simulink library "avl2DLiftingBdy_cl"  (R2018b)
settings: Solver=VariableStepAuto  StartTime=0.0  StopTime=10.0  RelTol=1e-3
values from neighbouring files (symbols this model uses):
  Bref = 1    [avl2DLiftingBdy_ts.m]
  Cref = 1    [avl2DLiftingBdy_ts.m]
  grav = 9.81    [avl2DLiftingBdy_ts.m]
  mass = 10    [avl2DLiftingBdy_ts.m]
  Rcb_cm = [0;0;0.1]    [avl2DLiftingBdy_ts.m]
  rho_fluid = 1    [avl2DLiftingBdy_ts.m]
  Sref = 1    [avl2DLiftingBdy_ts.m]
  vol = 20    [avl2DLiftingBdy_ts.m]
undefined symbols (not defined in the file or in its folder): CDtot_2D_Tbl, class_thr, CLtot_2D_Tbl, Cltot_2D_Tbl, Cmtot_2D_Tbl, Cntot_2D_Tbl, ini_euler, ini_O_Vcm_o, ini_OwB, ini_Rcm_o, k_CS_gain, MI, turbine
libraries: BdyFrameGravForce_ul x1, avlAerodynamics2D x1, bdyFrameBuoyFnM_ul x1, calcTetherEndNodesStates x1, simpleDragTurbine_ul x1, sixDoFDynamics_ul x1, sumTetherForcesAndMoments_ul x1
settings Model: Creator=Ayaz  LastModifiedBy=Ayaz

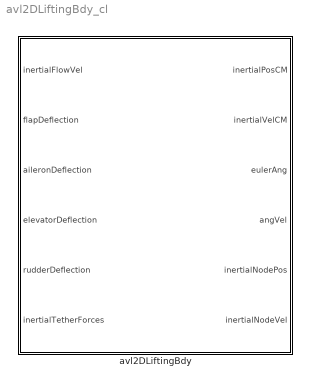
== system avl2DLiftingBdy_cl ==
  avl2DLiftingBdy : Subsystem  mask{M=mass, J=MI, vol=vol, Rcb_cm=Rcb_cm, turb_struct=turbine, thr_struct=class_thr, g=grav, rho_fluid=rho_fluid, initPos=ini_Rcm_o, initVel=ini_O_Vcm_o, initEulAngs=ini_euler, initAngVel=ini_OwB, CLTable=CLtot_2D_Tbl, CDTable=CDtot_2D_Tbl, CMxTable=Cltot_2D_Tbl, CMyTable=Cmtot_2D_Tbl, CMzTable=Cntot_2D_Tbl, CsGainMatrix=k_CS_gain, CRef=Cref, BRef=Bref, SRef=Sref}
      mask prompts: M "Mass"; J "Inertia matrix"; vol "Body volume"; Rcb_cm "Center of buoyamcy vector"; turb_struct "Turbines structure"; thr_struct "Tether class variable name"; g "Gravitational acceleration"; rho_fluid "Fluid density"; initPos "Initial position"; initVel "Initial velocity"; initEulAngs "Initial Euler Angles"; initAngVel "Initial Angular Velocity Vec"; CLTable "CL lookup table object"; CDTable "CD lookup table object"; CMxTable "CMx lookup table object"; CMyTable "CMy lookup table object"; CMzTable "CMz lookup table object"; CsGainMatrix "Control surface gain matrix"; CRef "Pitch Moment Reference Length (AVL Cref)"; BRef "Roll & Yaw Moment Reference Length (AVL Bref)"; SRef "Ref area (AVL Sref)"
      mask TypeOptions M: BdyFrameGravForce/M | sixDoFDynamics1/M
      mask TypeOptions J: sixDoFDynamics1/J
      mask TypeOptions vol: bdyFrameBuoyForceAndMoment/vol
      mask TypeOptions Rcb_cm: bdyFrameBuoyForceAndMoment/Rcb_cm
      mask TypeOptions turb_struct: simpleDragTurbine/turb_struct
      mask TypeOptions thr_struct: calcTetherEndNodesStates/thr_struct | sumTetherForcesAndMoments/thr_struct
      mask TypeOptions g: BdyFrameGravForce/g | bdyFrameBuoyForceAndMoment/g
      mask TypeOptions rho_fluid: avlAerodynamics2D/rho_fluid | bdyFrameBuoyForceAndMoment/rho_fluid | simpleDragTurbine/rho_fluid
      mask TypeOptions initPos: sixDoFDynamics1/initPos
      mask TypeOptions initVel: sixDoFDynamics1/initVel
      mask TypeOptions initEulAngs: sixDoFDynamics1/initEulAngs
      mask TypeOptions initAngVel: sixDoFDynamics1/initAngVel
      mask TypeOptions CLTable: avlAerodynamics2D/CLTable
      mask TypeOptions CDTable: avlAerodynamics2D/CDTable
      mask TypeOptions CMxTable: avlAerodynamics2D/CMxTable
      mask TypeOptions CMyTable: avlAerodynamics2D/CMyTable
      mask TypeOptions CMzTable: avlAerodynamics2D/CMzTable
      mask TypeOptions CsGainMatrix: avlAerodynamics2D/CsGainMatrix
      mask TypeOptions CRef: avlAerodynamics2D/CRef
      mask TypeOptions BRef: avlAerodynamics2D/BRef
      mask TypeOptions SRef: avlAerodynamics2D/SRef
      mask DialogControl Container20 Prompt: Parameters
      mask DialogControl ParameterGroupVar Prompt: Physical Parameters
      mask DialogControl Container24 Prompt: Environment
      mask DialogControl Container25 Prompt: Initial conditions
      mask DialogControl Container7 Prompt: AVL

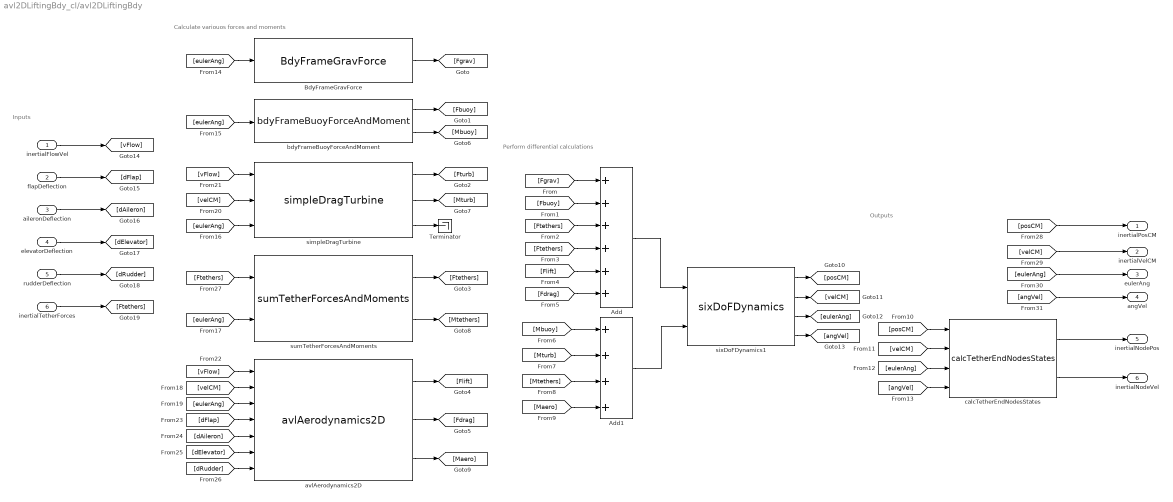
== system avl2DLiftingBdy_cl/avl2DLiftingBdy ==
  note: Outputs
  note: Inputs
  note: Calculate variouos forces and moments
  note: Perform differential calculations
  inertialFlowVel : Inport
  flapDeflection : Inport  Port=2
  aileronDeflection : Inport  Port=3
  elevatorDeflection : Inport  Port=4
  rudderDeflection : Inport  Port=5
  inertialTetherForces : Inport  Port=6
  Add : Sum  Inputs=++++++
  Add1 : Sum  Inputs=++++
  BdyFrameGravForce : BdyFrameGravForce_ul/BdyFrameGravForce  M=M  g=g
  Terminator : Terminator
  avlAerodynamics2D : avlAerodynamics2D/avlAerodynamics2D  CLTable=CLTable  CDTable=CDTable  CMxTable=CMxTable  CMyTable=CMyTable  CMzTable=CMzTable  CsGainMatrix=CsGainMatrix  CRef=CRef  BRef=BRef  SRef=SRef  rho_fluid=rho_fluid
  bdyFrameBuoyForceAndMoment : bdyFrameBuoyFnM_ul/bdyFrameBuoyForceAndMoment  vol=vol  rho_fluid=rho_fluid  g=g  Rcb_cm=Rcb_cm
  calcTetherEndNodesStates : calcTetherEndNodesStates/calcTetherEndNodesStates  thr_struct=thr_struct  attach_point=Lifting body
  simpleDragTurbine : simpleDragTurbine_ul/simpleDragTurbine  rho_fluid=rho_fluid  turb_struct=turb_struct
  sixDoFDynamics1 : sixDoFDynamics_ul/sixDoFDynamics  M=M  J=J  initPos=initPos  initVel=initVel  initEulAngs=initEulAngs  initAngVel=initAngVel
  sumTetherForcesAndMoments : sumTetherForcesAndMoments_ul/sumTetherForcesAndMoments  thr_struct=thr_struct  attach_point=Lifting body
  inertialPosCM : Outport
  inertialVelCM : Outport  Port=2
  eulerAng : Outport  Port=3
  angVel : Outport  Port=4
  inertialNodePos : Outport  Port=5
  inertialNodeVel : Outport  Port=6
  wires:
  [Mtethers] -> Add1/3
  [velCM] -> avlAerodynamics2D/2
  [angVel] -> calcTetherEndNodesStates/4
  [eulerAng] -> calcTetherEndNodesStates/3
  sixDoFDynamics1/4 -> [angVel]
  sixDoFDynamics1/3 -> [eulerAng]
  [posCM] -> calcTetherEndNodesStates/1
  sixDoFDynamics1/2 -> [velCM]
  [Mturb] -> Add1/2
  [eulerAng] -> sumTetherForcesAndMoments/2
  [eulerAng] -> bdyFrameBuoyForceAndMoment/1
  [eulerAng] -> BdyFrameGravForce/1
  [Mbuoy] -> Add1/1
  simpleDragTurbine/3 -> Terminator/1
  [Ftethers] -> Add/4
  avlAerodynamics2D/2 -> [Fdrag]
  Add1/1 -> sixDoFDynamics1/2
  avlAerodynamics2D/3 -> [Maero]
  [Fbuoy] -> Add/2
  avlAerodynamics2D/1 -> [Flift]
  sumTetherForcesAndMoments/1 -> [Ftethers]
  [velCM] -> calcTetherEndNodesStates/2
  [Maero] -> Add1/4
  [Ftethers] -> Add/3
  simpleDragTurbine/2 -> [Mturb]
  simpleDragTurbine/1 -> [Fturb]
  [Flift] -> Add/5
  Add/1 -> sixDoFDynamics1/1
  bdyFrameBuoyForceAndMoment/2 -> [Mbuoy]
  [eulerAng] -> avlAerodynamics2D/3
  BdyFrameGravForce/1 -> [Fgrav]
  [Fdrag] -> Add/6
  [Fgrav] -> Add/1
  sumTetherForcesAndMoments/2 -> [Mtethers]
  bdyFrameBuoyForceAndMoment/1 -> [Fbuoy]
  [eulerAng] -> simpleDragTurbine/3
  [velCM] -> simpleDragTurbine/2
  sixDoFDynamics1/1 -> [posCM]
  inertialFlowVel/1 -> [vFlow]
  [vFlow] -> simpleDragTurbine/1
  [vFlow] -> avlAerodynamics2D/1
  rudderDeflection/1 -> [dRudder]
  elevatorDeflection/1 -> [dElevator]
  aileronDeflection/1 -> [dAileron]
  flapDeflection/1 -> [dFlap]
  [dFlap] -> avlAerodynamics2D/4
  [dAileron] -> avlAerodynamics2D/5
  [dElevator] -> avlAerodynamics2D/6
  [dRudder] -> avlAerodynamics2D/7
  inertialTetherForces/1 -> [Ftethers]
  [Ftethers] -> sumTetherForcesAndMoments/1
  [posCM] -> inertialPosCM/1
  [velCM] -> inertialVelCM/1
  [eulerAng] -> eulerAng/1
  [angVel] -> angVel/1
  calcTetherEndNodesStates/2 -> inertialNodeVel/1
  calcTetherEndNodesStates/1 -> inertialNodePos/1
